simulink model "Controller"  (R2017a)
settings: Solver=FixedStepAuto  StartTime=0.0  StopTime=10000  FixedStep=200  MaxStep=4.0  MinStep=.001  RelTol=1e-6
undefined symbols (not defined in the file or in its folder): Klqr
libraries: vrlib x2
settings Model: Creator=armen  LastModifiedBy=armen
settings OptimizationCC: DefaultParameterBehavior=Inlined  UseDivisionForNetSlopeComputation=on  UseFloatMulNetSlope=on  InlineInvariantSignals=on  PassReuseOutputArgsAs=Individual arguments  ZeroExternalMemoryAtStartup=off  ZeroInternalMemoryAtStartup=off  NoFixptDivByZeroProtection=on  EfficientFloat2IntCast=on  LifeSpan=1
settings DebuggingCC: ParameterTunabilityLossMsg=error  FrameProcessingCompatibilityMsg=none
settings SFSimCC: MATLABDynamicMemAlloc=off
settings RTWCC: SystemTargetFile=ert.tlc  TLCOptions=-aAlwaysIncludeCustomSrc=1  GenCodeOnly=on  PackageGeneratedCodeAndArtifacts=on  PackageName=controller  TemplateMakefile=RTW.MSVCBuild  Description=Create Visual C/C++ Solution File for Embedded Coder  GenerateReport=on  IncludeHyperlinkInReport=on  LaunchReport=on  TargetLang=C++  GenerateTraceInfo=on  GenerateTraceReport=on  GenerateTraceReportSl=on  GenerateTraceReportSf=on  GenerateTraceReportEml=on
settings CodeAppCC: ForceParamTrailComments=on  IgnoreCustomStorageClasses=off  OperatorAnnotations=on  SimulinkDataObjDesc=on  SFDataObjDesc=on  MATLABFcnDesc=on  CustomSymbolStrGlobalVar=rt$N$M  CustomSymbolStrType=$N$M  CustomSymbolStrFcn=$N$M$F  CustomSymbolStrMacro=$N$M  InsertBlockDesc=on  MATLABSourceComments=on
settings ERTTargetCC: TargetLangStandard=C++03 (ISO)  GenerateSampleERTMain=on  IncludeMdlTerminateFcn=off  CombineSignalStateStructs=on  SupportAbsoluteTime=off  MultiInstanceERTCode=on  CodeInterfacePackaging=C++ class  SupportComplex=off  SupportContinuousTime=on  InlinedParameterPlacement=NonHierarchical  RootIOFormat=Structure reference  ERTCustomFileTemplate=example_file_process.tlc  ERTFilePackagingFormat=CompactWithDataFile

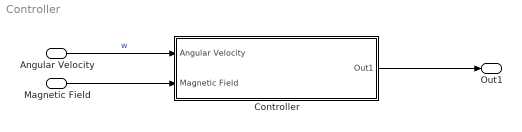
== system Controller ==
  Angular Velocity : Inport  OutDataTypeStr=double  PortDimensions=3  SampleTime=[-1 0]  Interpolate=off
  Magnetic Field : Inport  Port=2  OutDataTypeStr=double  PortDimensions=3  SampleTime=[-1 0]  Interpolate=off
  Controller : Subsystem  Tag=starshotsimv4p3lqrproto  TreatAsAtomicUnit=on
      settings: RTWSystemCode=Inline
  Out1 : Outport  OutDataTypeStr=double  PortDimensions=3  SampleTime=[-1 0]
  wires:
  Angular Velocity/1 -> Controller/1(Angular Velocity)  "w"
  Magnetic Field/1 -> Controller/2(Magnetic Field)
  Controller/1(Out1) -> Out1/1

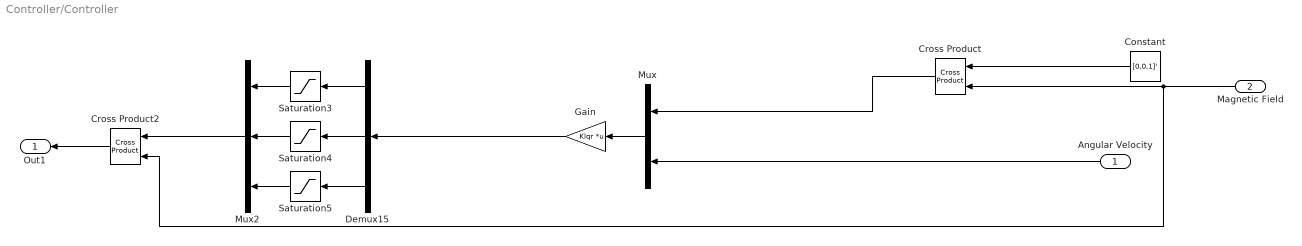
== system Controller/Controller ==
  Angular Velocity : Inport
  Magnetic Field : Inport  Port=2
  Constant : Constant  Value=[0,0,1]'
  Cross Product : vrlib/Utilities/Cross Product
      settings: SourceProductBaseCode=VR
  Cross Product2 : vrlib/Utilities/Cross Product
      settings: SourceProductBaseCode=VR
  Demux15 : Demux  Outputs=3
  Gain : Gain  Gain=Klqr  Multiplication=Matrix(K*u)
  Mux : Mux  Inputs=2
  Mux2 : Mux  Inputs=3
  Saturation3 : Saturate  UpperLimit=1.3  LowerLimit=-1.3
  Saturation4 : Saturate  UpperLimit=1.3  LowerLimit=-1.3
  Saturation5 : Saturate  UpperLimit=1.3  LowerLimit=-1.3
  Out1 : Outport
  wires:
  Constant/1 -> Cross Product/1
  Gain/1 -> Demux15/1
  Mux/1 -> Gain/1
  Angular Velocity/1 -> Mux/2
  Cross Product/1 -> Mux/1
  Magnetic Field/1 -> Cross Product/2, Cross Product2/2
  Mux2/1 -> Cross Product2/1
  Demux15/3 -> Saturation5/1
  Demux15/1 -> Saturation3/1
  Saturation5/1 -> Mux2/3
  Saturation3/1 -> Mux2/1
  Demux15/2 -> Saturation4/1
  Saturation4/1 -> Mux2/2
  Cross Product2/1 -> Out1/1
